simulink model "Shanthan_Heeirthan_EE469S3D_R45 (1)"  (R2023a)
settings: Solver=FixedStepDiscrete  StartTime=0.0  StopTime=120  FixedStep=dt0  RelTol=1e-3  EnableMultiTasking=on
PostLoadFcn:
  | %Set the size for the model
  | set_param(gcs,'Location',[10 10 1270 970])
  | %Set the zoom factor for the model
  | set_param(gcs,'ZoomFactor','100')
InitFcn:
  | tic
  | % Students Add call to their M-file HERE
  | Shanthan_Heeirthan_EE460_Final
  | INIT_S3D_01
StartFcn:
  | tend0=toc;
  | tic;
StopFcn:
  | tend=toc;
  | disp(['Simulation time = ' num2str(tout(end)) ' sec'])
  | disp(['Real time = ' num2str(tend) ' sec'])
  | title('DONE')
  | SCORE=round((max(0,120-tout(end)-tend0))*4+10*(40-FuelBurned)+sum(100*double(PDONE)-100*double(PDONE<.5)));
  | PlotS3D(PlotInput);
  | text(15,22,['S: ' num2str(SCORE)]);
values from neighbouring files (symbols this model uses):
  A = [0 1 0 0 0 0 ... (first row only)    [Shanthan_Heeirthan_EE460_Final (1).m]
  B = [0 0 0 ... (first row only)    [Shanthan_Heeirthan_EE460_Final (1).m]
  bm = [1 1 -1 -1 0 0 0 0; 0 0 0 0 -1 1 1 -1; -1 1 -1 1 3 -3 3 -3]    [Shanthan_Heeirthan_EE460_Final (1).m]
  C = [1 0 0 0 0 0 ... (first row only)    [Shanthan_Heeirthan_EE460_Final (1).m]
  D = [0 0 0 ... (first row only)    [Shanthan_Heeirthan_EE460_Final (1).m]
  Denchptheta = TFchptheta.Den{1}    [Shanthan_Heeirthan_EE460_Final (1).m]
  Denchpxy = TFchpxy.Den{1}    [Shanthan_Heeirthan_EE460_Final (1).m]
  Denclptheta = TFclptheta.Den{1}    [Shanthan_Heeirthan_EE460_Final (1).m]
  Denclpxy = TFclpxy.Den{1}    [Shanthan_Heeirthan_EE460_Final (1).m]
  Denlp = TFlp.Den{1}    [Shanthan_Heeirthan_EE460_Final (1).m]
  Kd = 2.1+0    (= 2.1)    [Shanthan_Heeirthan_EE460_Final (1).m]
  Ki = 0.0001    [Shanthan_Heeirthan_EE460_Final (1).m]
  Kp = 1.1+0.2    (= 1.3)    [Shanthan_Heeirthan_EE460_Final (1).m]
  L = place(A',C',ep)'    [Shanthan_Heeirthan_EE460_Final (1).m]
  Numchptheta = TFchptheta.Num{1}    [Shanthan_Heeirthan_EE460_Final (1).m]
  Numchpxy = TFchpxy.Num{1}    [Shanthan_Heeirthan_EE460_Final (1).m]
  Numclptheta = TFclptheta.Num{1}    [Shanthan_Heeirthan_EE460_Final (1).m]
  Numclpxy = TFclpxy.Num{1}    [Shanthan_Heeirthan_EE460_Final (1).m]
  Numlp = TFlp.Num{1}    [Shanthan_Heeirthan_EE460_Final (1).m]
  Pnewdata = [LVL.P1 LVL.P2 LVL.P3 LVL.P4]    [Shanthan_Heeirthan_EE460_Final (1).m]
  Sconfig = 1    [Shanthan_Heeirthan_EE460_Final (1).m]
  TFP1 = 2    [Shanthan_Heeirthan_EE460_Final (1).m]
  TFP1z = 1    [Shanthan_Heeirthan_EE460_Final (1).m]
  TFP2 = 2    [Shanthan_Heeirthan_EE460_Final (1).m]
  TFP2z = 1    [Shanthan_Heeirthan_EE460_Final (1).m]
  TFP3 = 2    [Shanthan_Heeirthan_EE460_Final (1).m]
  TFP3z = 1    [Shanthan_Heeirthan_EE460_Final (1).m]
  TFP4 = 2    [Shanthan_Heeirthan_EE460_Final (1).m]
  TFP4z = 1    [Shanthan_Heeirthan_EE460_Final (1).m]
  wcf = 2    [Shanthan_Heeirthan_EE460_Final (1).m]
  wcft = 10    [Shanthan_Heeirthan_EE460_Final (1).m]
undefined symbols (not defined in the file or in its folder): d2r, DiscIntNeverNeededParam, dt, dt0, fr, HM_S, HM_U, J, Jbase, JC0, L13, L24, LVL, M, M1, M2, M3, M4, mdti, Pdata, PTvec, r2d, SLIM, SQ, SSF, TOLdata, ULIM
libraries: simulink x85, aerolibanimutils x1, matrix_library x1
(part 2 of 7)

== system Shanthan_Heeirthan_EE469S3D_R45 (1)/S3D_Plant/Sensors/CASE1 ==
  X : Inport
  Action Port : ActionPort  ActionPortLabel=case [ 1 ]:
  Constant2 : Constant  Value=SSF  SampleTime=dt0
  Gain : Gain
  Mux{,1..3} (4 alike) : Mux  Inputs=3
  Product : Product
  THTaccel : Subsystem
  THTpos1 : Subsystem
  THTvel : Subsystem
  Xaccel : Subsystem
  Xpos1 : Subsystem
  Xvel : Subsystem
  Yaccel : Subsystem
  Ypos1 : Subsystem
  Yvel : Subsystem
  Out1 : Outport
  wires:
  Constant2/1 -> Product/2
  Product/1 -> Gain/1
  Mux3/1 -> Product/1
  Gain/1 -> Out1/1
  THTaccel/1(thtddt1) -> Mux2/3
  THTvel/1(thtdt1) -> Mux2/2
  THTpos1/1(tht1) -> Mux2/1
  Mux2/1 -> Mux3/3
  Yaccel/1(yddt1) -> Mux1/3
  Yvel/1(ydt1) -> Mux1/2
  Ypos1/1(y1) -> Mux1/1
  Mux1/1 -> Mux3/2
  Mux/1 -> Mux3/1
  Xaccel/1(xddt1) -> Mux/3
  Xpos1/1(x1) -> Mux/1
  Xvel/1(xdt1) -> Mux/2
  X/1 -> Xpos1/1(X), Xvel/1(X), Xaccel/1(X), Ypos1/1(X), Yvel/1(X), Yaccel/1(X), THTpos1/1(X), THTvel/1(X), THTaccel/1(X)

== system Shanthan_Heeirthan_EE469S3D_R45 (1)/S3D_Plant/Sensors/CASE2 ==
  X : Inport
  Action Port : ActionPort  ActionPortLabel=case [ 2 ]:
  Constant2 : Constant  Value=SSF([1 1 2 4 4 5 7 7 8])  SampleTime=dt0
  Gain : Gain
  Mux{,1..3} (4 alike) : Mux  Inputs=3
  Product : Product
  THTpos1 : Subsystem
  THTpos2 : Subsystem
  THTvel : Subsystem
  Xpos1 : Subsystem
  Xpos2 : Subsystem
  Xvel : Subsystem
  Ypos1 : Subsystem
  Ypos2 : Subsystem
  Yvel : Subsystem
  Out1 : Outport
  wires:
  Constant2/1 -> Product/2
  Product/1 -> Gain/1
  Mux3/1 -> Product/1
  Gain/1 -> Out1/1
  X/1 -> THTvel/1(X), THTpos2/1(X), THTpos1/1(X), Yvel/1(X), Ypos2/1(X), Ypos1/1(X), Xvel/1(X), Xpos2/1(X), Xpos1/1(X)
  Xpos2/1(x1) -> Mux/2
  Xpos1/1(x1) -> Mux/1
  Xvel/1(xdt1) -> Mux/3
  Mux/1 -> Mux3/1
  Mux1/1 -> Mux3/2
  Ypos1/1(y1) -> Mux1/1
  Ypos2/1(y1) -> Mux1/2
  Yvel/1(ydt1) -> Mux1/3
  Mux2/1 -> Mux3/3
  THTpos1/1(tht1) -> Mux2/1
  THTpos2/1(tht1) -> Mux2/2
  THTvel/1(thtdt1) -> Mux2/3

== system Shanthan_Heeirthan_EE469S3D_R45 (1)/S3D_Plant/Sensors/CASE3 ==
  X : Inport
  Action Port : ActionPort  ActionPortLabel=default:
  Constant2 : Constant  Value=SSF([1 1 1 4 4 4 7 7 7])  SampleTime=dt0
  Gain : Gain
  Mux{,1..3} (4 alike) : Mux  Inputs=3
  Product : Product
  THTpos1 : Subsystem
  THTpos2 : Subsystem
  THTpos3 : Subsystem
  Xpos1 : Subsystem
  Xpos2 : Subsystem
  Xpos3 : Subsystem
  Ypos1 : Subsystem
  Ypos2 : Subsystem
  Ypos3 : Subsystem
  Out1 : Outport
  wires:
  Constant2/1 -> Product/2
  Product/1 -> Gain/1
  Mux3/1 -> Product/1
  Gain/1 -> Out1/1
  THTpos3/1(tht1) -> Mux2/3
  THTpos2/1(tht1) -> Mux2/2
  THTpos1/1(tht1) -> Mux2/1
  Mux2/1 -> Mux3/3
  Ypos3/1(y1) -> Mux1/3
  Ypos2/1(y1) -> Mux1/2
  Ypos1/1(y1) -> Mux1/1
  Mux1/1 -> Mux3/2
  Mux/1 -> Mux3/1
  Xpos3/1(xddt1) -> Mux/3
  Xpos1/1(x1) -> Mux/1
  Xpos2/1(xdt1) -> Mux/2
  X/1 -> Xpos1/1(X), Ypos1/1(X), THTpos1/1(X), THTpos2/1(X), THTpos3/1(X), Ypos3/1(X), Ypos2/1(X), Xpos3/1(X), Xpos2/1(X)

== system Shanthan_Heeirthan_EE469S3D_R45 (1)/S3D_Plant/Sensors/ConvertINT16 ==
  SDouble : Inport
  Bus Creator : BusCreator  Inputs=9
  Data Type Conversion{,1..8} (9 alike) : DataTypeConversion  OutDataTypeStr=int16  SampleTime=dt0  SaturateOnIntegerOverflow=off  RndMeth=Floor
  Demux : Demux  Outputs=9
  INT16 : Outport
  wires:
  Data Type Conversion8/1 -> Bus Creator/9  "Sensor9"
  Data Type Conversion7/1 -> Bus Creator/8  "Sensor8"
  Data Type Conversion6/1 -> Bus Creator/7  "Sensor7"
  Data Type Conversion5/1 -> Bus Creator/6  "Sensor6"
  Data Type Conversion4/1 -> Bus Creator/5  "Sensor5"
  Data Type Conversion3/1 -> Bus Creator/4  "Sensor4"
  Data Type Conversion2/1 -> Bus Creator/3  "Sensor3"
  Demux/5 -> Data Type Conversion4/1
  Demux/3 -> Data Type Conversion2/1
  Demux/6 -> Data Type Conversion5/1
  Demux/4 -> Data Type Conversion3/1
  Demux/9 -> Data Type Conversion8/1
  Demux/7 -> Data Type Conversion6/1
  Demux/8 -> Data Type Conversion7/1
  SDouble/1 -> Demux/1
  Data Type Conversion1/1 -> Bus Creator/2  "Sensor2"
  Bus Creator/1 -> INT16/1  "INT16"
  Demux/1 -> Data Type Conversion/1
  Demux/2 -> Data Type Conversion1/1
  Data Type Conversion/1 -> Bus Creator/1  "Sensor1"

== system Shanthan_Heeirthan_EE469S3D_R45 (1)/S3D_Plant/Sensors/HealthMonitoring ==
  SensorValues : Inport
  Bus Creator1 : BusCreator  Inputs=18
  Bus Selector1 : BusSelector  OutputSignals=Sensor1,Sensor2,Sensor3,Sensor4,Sensor5,Sensor6,Sensor7,Sensor8,Sensor9
  Bus Selector2 : BusSelector  OutputSignals=Sensor1,Sensor2,Sensor3,Sensor4,Sensor5,Sensor6,Sensor7,Sensor8,Sensor9
  Subsystem : Subsystem
  Subsystem1 : Subsystem
  Subsystem2 : Subsystem
  Subsystem3 : Subsystem
  Subsystem4 : Subsystem
  Subsystem5 : Subsystem
  Subsystem6 : Subsystem
  Subsystem7 : Subsystem
  Subsystem8 : Subsystem
  Sensors : Outport
  wires:
  Bus Creator1/1 -> Sensors/1  "Sensors"
  Bus Selector2/4 -> Bus Creator1/4  "<Sensor4>"
  Bus Selector2/8 -> Bus Creator1/8  "<Sensor8>"
  Bus Selector2/6 -> Bus Creator1/6  "<Sensor6>"
  Bus Selector2/5 -> Bus Creator1/5  "<Sensor5>"
  Bus Selector2/3 -> Bus Creator1/3  "<Sensor3>"
  Bus Selector2/9 -> Bus Creator1/9  "<Sensor9>"
  Bus Selector2/2 -> Bus Creator1/2  "<Sensor2>"
  Bus Selector2/1 -> Bus Creator1/1  "<Sensor1>"
  Bus Selector2/7 -> Bus Creator1/7  "<Sensor7>"
  SensorValues/1 -> Bus Selector1/1, Bus Selector2/1
  Subsystem/1(Out1) -> Bus Creator1/10  "S1fail"
  Bus Selector1/8 -> Subsystem7/1(In1)  "<Sensor8>"
  Bus Selector1/3 -> Subsystem2/1(In1)  "<Sensor3>"
  Bus Selector1/7 -> Subsystem6/1(In1)  "<Sensor7>"
  Bus Selector1/2 -> Subsystem1/1(In1)  "<Sensor2>"
  Subsystem2/1(Out1) -> Bus Creator1/12  "S3fail"
  Subsystem1/1(Out1) -> Bus Creator1/11  "S2fail"
  Bus Selector1/6 -> Subsystem5/1(In1)  "<Sensor6>"
  Subsystem3/1(Out1) -> Bus Creator1/13  "S4fail"
  Bus Selector1/4 -> Subsystem3/1(In1)  "<Sensor4>"
  Bus Selector1/5 -> Subsystem4/1(In1)  "<Sensor5>"
  Bus Selector1/9 -> Subsystem8/1(In1)  "<Sensor9>"
  Subsystem5/1(Out1) -> Bus Creator1/15  "S6fail"
  Subsystem4/1(Out1) -> Bus Creator1/14  "S5fail"
  Subsystem6/1(Out1) -> Bus Creator1/16  "S7fail"
  Subsystem8/1(Out1) -> Bus Creator1/18  "S9fail"
  Subsystem7/1(Out1) -> Bus Creator1/17  "S8fail"
  Bus Selector1/1 -> Subsystem/1(In1)  "<Sensor1>"

== system Shanthan_Heeirthan_EE469S3D_R45 (1)/S3D_Plant/ThrusterValues/FailModes ==
  Ucmd : Inport
  MP : Inport  Port=2
  Bus Creator : BusCreator  Inputs=10
  Ufail1 : Subsystem  mask{Udx=1, Tank=1}
      mask prompts: Udx "Input Index of U (1-8)"; Tank "Input Fuel Tank (1-4)"
  Ufail10 : Subsystem  mask{Udx=10, Tank=1}
      mask prompts: Udx "Input Index of U (1-8)"; Tank "Input Fuel Tank (1-4)"
  Ufail2 : Subsystem  mask{Udx=2, Tank=2}
      mask prompts: Udx "Input Index of U (1-8)"; Tank "Input Fuel Tank (1-4)"
  Ufail3 : Subsystem  mask{Udx=3, Tank=3}
      mask prompts: Udx "Input Index of U (1-8)"; Tank "Input Fuel Tank (1-4)"
  Ufail4 : Subsystem  mask{Udx=4, Tank=4}
      mask prompts: Udx "Input Index of U (1-8)"; Tank "Input Fuel Tank (1-4)"
  Ufail5 : Subsystem  mask{Udx=5, Tank=1}
      mask prompts: Udx "Input Index of U (1-8)"; Tank "Input Fuel Tank (1-4)"
  Ufail6 : Subsystem  mask{Udx=6, Tank=2}
      mask prompts: Udx "Input Index of U (1-8)"; Tank "Input Fuel Tank (1-4)"
  Ufail7 : Subsystem  mask{Udx=7, Tank=3}
      mask prompts: Udx "Input Index of U (1-8)"; Tank "Input Fuel Tank (1-4)"
  Ufail8 : Subsystem  mask{Udx=8, Tank=4}
      mask prompts: Udx "Input Index of U (1-8)"; Tank "Input Fuel Tank (1-4)"
  Ufail9 : Subsystem  mask{Udx=9, Tank=1}
      mask prompts: Udx "Input Index of U (1-8)"; Tank "Input Fuel Tank (1-4)"
  U : Outport
  wires:
  Bus Creator/1 -> U/1  "U"
  Ufail7/1(Uout) -> Bus Creator/7  "U7"
  Ufail6/1(Uout) -> Bus Creator/6  "U6"
  Ufail8/1(Uout) -> Bus Creator/8  "U8"
  Ufail9/1(Uout) -> Bus Creator/9  "U9"
  Ufail10/1(Uout) -> Bus Creator/10  "U10"
  Ufail5/1(Uout) -> Bus Creator/5  "U5"
  Ufail4/1(Uout) -> Bus Creator/4  "U4"
  Ufail3/1(Uout) -> Bus Creator/3  "U3"
  Ufail2/1(Uout) -> Bus Creator/2  "U2"
  Ufail1/1(Uout) -> Bus Creator/1  "U1"
  MP/1 -> Ufail1/2(MP), Ufail3/2(MP), Ufail4/2(MP), Ufail8/2(MP), Ufail7/2(MP), Ufail6/2(MP), Ufail5/2(MP), Ufail2/2(MP)
  Ucmd/1 -> Ufail1/1(Uin), Ufail4/1(Uin), Ufail9/1(Uin), Ufail10/1(Uin), Ufail8/1(Uin), Ufail7/1(Uin), Ufail6/1(Uin), Ufail5/1(Uin), Ufail3/1(Uin), Ufail2/1(Uin)

== system Shanthan_Heeirthan_EE469S3D_R45 (1)/S3D_Plant/ThrusterValues/HealthMonitoring ==
  Uvalues : Inport
  UCMD : Inport  Port=2
  Bus Creator2 : BusCreator  Inputs=20
  Bus Selector10 : BusSelector  OutputSignals=U1,U2,U3,U4,U5,U6,U7,U8,U9,U10
  Bus Selector11 : BusSelector  OutputSignals=U1fail,U2fail,U3fail,U4fail,U5fail,U6fail,U7fail,U8fail,U9fail,U10fail
  DetectFailures : Subsystem
  U : Outport
  wires:
  Bus Selector10/1 -> Bus Creator2/1  "<U1>"
  Bus Selector10/2 -> Bus Creator2/2  "<U2>"
  Bus Selector10/9 -> Bus Creator2/9  "<U9>"
  Bus Selector10/5 -> Bus Creator2/5  "<U5>"
  Bus Selector10/3 -> Bus Creator2/3  "<U3>"
  Bus Selector10/6 -> Bus Creator2/6  "<U6>"
  Bus Selector10/7 -> Bus Creator2/7  "<U7>"
  Bus Selector10/8 -> Bus Creator2/8  "<U8>"
  Bus Selector10/4 -> Bus Creator2/4  "<U4>"
  Bus Selector10/10 -> Bus Creator2/10  "<U10>"
  Bus Creator2/1 -> U/1  "U"
  Bus Selector11/1 -> Bus Creator2/11  "<U1fail>"
  Bus Selector11/2 -> Bus Creator2/12  "<U2fail>"
  Bus Selector11/3 -> Bus Creator2/13  "<U3fail>"
  Bus Selector11/4 -> Bus Creator2/14  "<U4fail>"
  Bus Selector11/5 -> Bus Creator2/15  "<U5fail>"
  Bus Selector11/6 -> Bus Creator2/16  "<U6fail>"
  Bus Selector11/7 -> Bus Creator2/17  "<U7fail>"
  Bus Selector11/8 -> Bus Creator2/18  "<U8fail>"
  Bus Selector11/9 -> Bus Creator2/19  "<U9fail>"
  Bus Selector11/10 -> Bus Creator2/20  "<U10fail>"
  UCMD/1 -> DetectFailures/2(UCMD)
  Uvalues/1 -> DetectFailures/1(Uvalues), Bus Selector10/1
  DetectFailures/1(Out2) -> Bus Selector11/1

== system Shanthan_Heeirthan_EE469S3D_R45 (1)/control_law/CMD/CMDprocess ==
  Y_IN : Inport
  Bus Selector : BusSelector  OutputSignals=Y_IN_sens.X1_m,Y_IN_sens.Y_m  OutputAsBus=on
  CommandTypes : Subsystem
  Constant : Constant
  Constant3 : Constant  Value=Pnewdata
  Selector1 : Selector  NumberOfDimensions=2  InputPortWidth=3  IndexOptions=Select all,Index vector (port)  Indices=[1 3],1  OutputSizes=1,1
  CMD : Outport
  wires:
  Constant3/1 -> Selector1/1  "Pdata"
  Y_IN/1 -> Bus Selector/1
  Selector1/1 -> CommandTypes/1(Pdata)  "CMDS"
  CommandTypes/1(CMDS) -> CMD/1
  Constant/1 -> Selector1/2, CommandTypes/2(Point)  "Point"
  Bus Selector/1 -> CommandTypes/3(Sensed)  "Sensed"

== system Shanthan_Heeirthan_EE469S3D_R45 (1)/control_law/InputDataConditioning/SensorConditioning ==
  Y_BUS : Inport
  Bus Creator : BusCreator  Inputs=9
  Bus Selector : BusSelector  OutputSignals=S1fail,S2fail,S3fail,Sensor1,Sensor2,Sensor3  OutputAsBus=on
  Bus Selector1 : BusSelector  OutputSignals=S4fail,S5fail,S6fail,Sensor4,Sensor5,Sensor6  OutputAsBus=on
  Bus Selector2 : BusSelector  OutputSignals=Sensor7,Sensor8,Sensor9,S7fail,S8fail,S9fail  OutputAsBus=on
  JustX : Subsystem
  JustY : Subsystem
  JustZ : Subsystem
  Y_sens : Outport
  wires:
  Y_BUS/1 -> Bus Selector2/1, Bus Selector/1, Bus Selector1/1
  Bus Selector/1 -> JustX/1(Xsens)  "Sensors"
  Bus Selector1/1 -> JustY/1(Ysens)  "Sensors"
  Bus Selector2/1 -> JustZ/1(Zsens)  "Sensors"
  JustX/1(xpos) -> Bus Creator/1  "X1_m"
  Bus Creator/1 -> Y_sens/1  "Y_IN_sens"
  JustX/2(xvel) -> Bus Creator/2  "X_mps"
  JustX/3(xacc) -> Bus Creator/3  "X_mps2"
  JustY/1(ypos) -> Bus Creator/4  "Y_m"
  JustY/2(yvel) -> Bus Creator/5  "Y_mps"
  JustY/3(yacc) -> Bus Creator/6  "Y_mps2"
  JustZ/1(thetapos) -> Bus Creator/7  "theta_deg"
  JustZ/2(thetavel) -> Bus Creator/8  "theta_degps"
  JustZ/3(thetaacc) -> Bus Creator/9  "theta_degps2"

== system Shanthan_Heeirthan_EE469S3D_R45 (1)/control_law/InputDataConditioning/xhatsel ==
  xhat : Inport
  Bus Creator1 : BusCreator  Inputs=6
  Demux : Demux  Outputs=6
  Gain : Gain  Gain=180/pi
  Gain1 : Gain  Gain=180/pi
  x_hat : Outport
  wires:
  xhat/1 -> Demux/1
  Demux/4 -> Bus Creator1/4  "y_vel_est_mps"
  Bus Creator1/1 -> x_hat/1  "x_hat"
  Demux/2 -> Bus Creator1/2  "x_vel_est_mps"
  Demux/3 -> Bus Creator1/3  "y_pos_est_m"
  Demux/1 -> Bus Creator1/1  "x_pos_est_m"
  Demux/6 -> Gain1/1  "theta_vel_est_radps"
  Gain1/1 -> Bus Creator1/6  "theta_vel_est_degps"
  Demux/5 -> Gain/1  "theta_pos_est_rad"
  Gain/1 -> Bus Creator1/5  "theta_pos_est_deg"

== system Shanthan_Heeirthan_EE469S3D_R45 (1)/control_law/Regulator/CompX ==
  Y_IN : Inport
  Bus Creator : BusCreator  Inputs=2
  Bus Selector : BusSelector  OutputSignals=Y_IN_sens.X1_m,Y_IN_sens.X_mps,Y_IN_sens.X_mps2
  Discrete Transfer Fcn : DiscreteTransferFcn  Numerator=Numclpxy  Denominator=Denclpxy  SampleTime=dt
  Discrete Transfer Fcn1 : DiscreteTransferFcn  Numerator=Numchpxy  Denominator=Denchpxy  SampleTime=dt
  Discrete Transfer Fcn2 : DiscreteTransferFcn  Numerator=Numchpxy  Denominator=Denchpxy  SampleTime=dt
  Gain : Gain  Gain=wcf
  Sum : Sum  Inputs=|++
  Sum1 : Sum  Inputs=|++
  X_filt : Outport
  wires:
  Y_IN/1 -> Bus Selector/1
  Bus Selector/1 -> Discrete Transfer Fcn/1  "<X1_m>"
  Bus Selector/2 -> Discrete Transfer Fcn1/1  "<X_mps>"
  Bus Selector/3 -> Discrete Transfer Fcn2/1  "<X_mps2>"
  Sum1/1 -> Bus Creator/2  "X_mps"
  Gain/1 -> Sum1/1
  Discrete Transfer Fcn/1 -> Sum/1
  Discrete Transfer Fcn1/1 -> Sum/2, Gain/1
  Discrete Transfer Fcn2/1 -> Sum1/2
  Sum/1 -> Bus Creator/1  "X1_m"
  Bus Creator/1 -> X_filt/1

== system Shanthan_Heeirthan_EE469S3D_R45 (1)/control_law/Regulator/CompY ==
  Y_IN : Inport
  Bus Creator : BusCreator  Inputs=2
  Bus Selector : BusSelector  OutputSignals=Y_IN_sens.Y_m,Y_IN_sens.Y_mps,Y_IN_sens.Y_mps2
  Discrete Transfer Fcn : DiscreteTransferFcn  Numerator=Numclpxy  Denominator=Denclpxy  SampleTime=dt
  Discrete Transfer Fcn1 : DiscreteTransferFcn  Numerator=Numchpxy  Denominator=Denchpxy  SampleTime=dt
  Discrete Transfer Fcn2 : DiscreteTransferFcn  Numerator=Numchpxy  Denominator=Denchpxy  SampleTime=dt
  Gain : Gain  Gain=wcf
  Sum : Sum  Inputs=|++
  Sum1 : Sum  Inputs=|++
  Y_filt : Outport
  wires:
  Bus Creator/1 -> Y_filt/1
  Sum/1 -> Bus Creator/1  "Y_m"
  Discrete Transfer Fcn2/1 -> Sum1/2
  Discrete Transfer Fcn1/1 -> Gain/1, Sum/2
  Discrete Transfer Fcn/1 -> Sum/1
  Gain/1 -> Sum1/1
  Sum1/1 -> Bus Creator/2  "Y_mps"
  Bus Selector/3 -> Discrete Transfer Fcn2/1  "<Y_mps2>"
  Bus Selector/2 -> Discrete Transfer Fcn1/1  "<Y_mps>"
  Bus Selector/1 -> Discrete Transfer Fcn/1  "<Y_m>"
  Y_IN/1 -> Bus Selector/1

== system Shanthan_Heeirthan_EE469S3D_R45 (1)/control_law/Regulator/Comptheta ==
  Y_IN : Inport
  Bus Creator : BusCreator  Inputs=2
  Bus Selector : BusSelector  OutputSignals=Y_IN_sens.theta_deg,Y_IN_sens.theta_degps,Y_IN_sens.theta_degps2
  Discrete Transfer Fcn : DiscreteTransferFcn  Numerator=Numclptheta  Denominator=Denclptheta  SampleTime=dt
  Discrete Transfer Fcn1 : DiscreteTransferFcn  Numerator=Numchptheta  Denominator=Denchptheta  SampleTime=dt
  Discrete Transfer Fcn2 : DiscreteTransferFcn  Numerator=Numchptheta  Denominator=Denchptheta  SampleTime=dt
  Gain : Gain  Gain=wcft
  Sum : Sum  Inputs=|++
  Sum1 : Sum  Inputs=|++
  theta_filt : Outport
  wires:
  Bus Creator/1 -> theta_filt/1
  Sum/1 -> Bus Creator/1  "theta_deg"
  Discrete Transfer Fcn2/1 -> Sum1/2
  Discrete Transfer Fcn1/1 -> Gain/1, Sum/2
  Discrete Transfer Fcn/1 -> Sum/1
  Gain/1 -> Sum1/1
  Sum1/1 -> Bus Creator/2  "theta_degps"
  Bus Selector/3 -> Discrete Transfer Fcn2/1  "<theta_degps2>"
  Bus Selector/2 -> Discrete Transfer Fcn1/1  "<theta_degps>"
  Bus Selector/1 -> Discrete Transfer Fcn/1  "<theta_deg>"
  Y_IN/1 -> Bus Selector/1

== system Shanthan_Heeirthan_EE469S3D_R45 (1)/control_law/Regulator/MassVariable ==
  Ulim : Inport
  Bus Creator : BusCreator  Inputs=10
  Bus to Vector : BusToVector
  Constant : Constant  Value=M
  Demux : Demux  Outputs=10
  Discrete-Time Integrator : DiscreteIntegrator  SampleTime=-1  ICPrevOutput=DiscIntNeverNeededParam  ICPrevScaledInput=DiscIntNeverNeededParam
  Gain : Gain  Gain=mdti
  Sum : Sum  Inputs=+
  Sum1 : Sum  Inputs=|+-
  Mass : Outport
  wires:
  Ulim/1 -> Demux/1
  Demux/1 -> Bus Creator/1  "U1cmd"
  Demux/2 -> Bus Creator/2  "U2cmd"
  Demux/3 -> Bus Creator/3  "U3cmd"
  Demux/4 -> Bus Creator/4  "U4cmd"
  Demux/5 -> Bus Creator/5  "U5cmd"
  Demux/6 -> Bus Creator/6  "U6cmd"
  Demux/7 -> Bus Creator/7  "U7cmd"
  Demux/8 -> Bus Creator/8  "U8cmd"
  Demux/9 -> Bus Creator/9  "U9cmd"
  Demux/10 -> Bus Creator/10  "U10cmd"
  Bus Creator/1 -> Bus to Vector/1
  Bus to Vector/1 -> Gain/1
  Gain/1 -> Discrete-Time Integrator/1  "mdot"
  Discrete-Time Integrator/1 -> Sum/1  "mchanged"
  Sum/1 -> Sum1/2
  Constant/1 -> Sum1/1  "realm"
  Sum1/1 -> Mass/1  "Mass"

== system Shanthan_Heeirthan_EE469S3D_R45 (1)/control_law/thrustercmd/CAcreator ==
  DCM : Inport
  U_lim : Inport  Port=2
  Bus Creator : BusCreator  Inputs=10
  Bus Creator1 : BusCreator  Inputs=8
  Bus Selector : BusSelector  OutputSignals=U1cmd,U2cmd,U3cmd,U4cmd,U5cmd,U6cmd,U7cmd,U8cmd
  Constant : Constant  Value=bm
  Demux1 : Demux  Outputs=10
  Matrix Multiply : Product  Multiplication=Matrix(*)
  Matrix Multiply1 : Product  Multiplication=Matrix(*)
  Transpose : Math  Operator=transpose
  CAout : Outport
  wires:
  Demux1/4 -> Bus Creator/4  "U4cmd"
  Bus Selector/5 -> Bus Creator1/5  "<U5cmd>"
  Demux1/7 -> Bus Creator/7  "U7cmd"
  Bus Selector/2 -> Bus Creator1/2  "<U2cmd>"
  Bus Selector/3 -> Bus Creator1/3  "<U3cmd>"
  Demux1/9 -> Bus Creator/9  "U9cmd"
  Demux1/5 -> Bus Creator/5  "U5cmd"
  Demux1/2 -> Bus Creator/2  "U2cmd"
  Demux1/1 -> Bus Creator/1  "U1cmd"
  Demux1/8 -> Bus Creator/8  "U8cmd"
  Bus Selector/4 -> Bus Creator1/4  "<U4cmd>"
  Demux1/10 -> Bus Creator/10  "U10cmd"
  Demux1/3 -> Bus Creator/3  "U3cmd"
  Bus Creator/1 -> Bus Selector/1  "Ulim"
  Bus Selector/7 -> Bus Creator1/7  "<U7cmd>"
  Bus Selector/1 -> Bus Creator1/1  "<U1cmd>"
  Demux1/6 -> Bus Creator/6  "U6cmd"
  Bus Selector/6 -> Bus Creator1/6  "<U6cmd>"
  Bus Selector/8 -> Bus Creator1/8  "<U8cmd>"
  U_lim/1 -> Demux1/1
  Constant/1 -> Matrix Multiply/1  "bm"
  Bus Creator1/1 -> Matrix Multiply/2  "Ulim"
  Matrix Multiply1/1 -> CAout/1  "CAout"
  Matrix Multiply/1 -> Matrix Multiply1/2  "CAout"
  DCM/1 -> Transpose/1
  Transpose/1 -> Matrix Multiply1/1

== system Shanthan_Heeirthan_EE469S3D_R45 (1)/control_law/thrustercmd/DCM ==
  Y_IN : Inport
  Bus Selector : BusSelector  OutputSignals=Y_IN_sens.theta_deg
  Constant : Constant  Value=[0 0 0;0 0 0;0 0 1]
  Cos : Trigonometry  Operator=cos
  Gain : Gain  Gain=pi/180
  Gain1 : Gain  Gain=[1 0 0; 0 1 0; 0 0 0]
  Gain2 : Gain  Gain=[0 -1 0;1 0 0;0 0 0]
  Sin : Trigonometry
  Sum : Sum  Inputs=|++
  Sum1 : Sum  Inputs=|++
  Transpose : Math  Operator=transpose
  IUR : Outport
  wires:
  Y_IN/1 -> Bus Selector/1
  Bus Selector/1 -> Gain/1  "<theta_deg>"
  Gain/1 -> Cos/1, Sin/1
  Cos/1 -> Gain1/1
  Sin/1 -> Gain2/1
  Gain1/1 -> Sum/1
  Gain2/1 -> Sum/2
  Sum/1 -> Sum1/1
  Constant/1 -> Sum1/2
  Sum1/1 -> Transpose/1
  Transpose/1 -> IUR/1

== system Shanthan_Heeirthan_EE469S3D_R45 (1)/control_law/thrustercmd/GenInverse ==
  Ufail : Inport
  Constant : Constant  Value=bm
  Constant2 : Constant  Value=bm
  Divide : Product  Inputs=/  Multiplication=Matrix(*)
  Divide1 : Product  Inputs=/  Multiplication=Matrix(*)
  Divide2 : Product  Inputs=/  Multiplication=Matrix(*)
  Gain : Gain  Gain=2
  Matrix Multiply{,1..3} (4 alike) : Product  Multiplication=Matrix(*)
  Transpose{,1..3} (4 alike) : Math  Operator=transpose
  WeightedMatrix : Subsystem
  ginv : Outport
  wires:
  WeightedMatrix/1(Weight) -> Transpose2/1, Transpose/1
  Transpose/1 -> Divide/1
  Constant/1 -> Matrix Multiply1/1, Transpose1/1
  Divide/1 -> Matrix Multiply/1
  Transpose1/1 -> Matrix Multiply/2
  Transpose2/1 -> Divide1/1
  Divide1/1 -> Matrix Multiply1/2
  Matrix Multiply1/1 -> Matrix Multiply2/1
  Matrix Multiply2/1 -> Divide2/1
  Matrix Multiply/1 -> Matrix Multiply3/1
  Divide2/1 -> Matrix Multiply3/2
  Constant2/1 -> Transpose3/1
  Transpose3/1 -> Matrix Multiply2/2
  Matrix Multiply3/1 -> Gain/1  "pinv"
  Gain/1 -> ginv/1  "ginv"
  Ufail/1 -> WeightedMatrix/1(Ufail)

== system Shanthan_Heeirthan_EE469S3D_R45 (1)/S3D_Plant/Comm/P1/DirectionCompensation2 ==
  In1 : Inport
  Compare To Constant : simulink/Logic and Bit Operations/Compare To Constant  relop=<=  const=pi  OutDataTypeStr=boolean
  Compare To Constant1 : simulink/Logic and Bit Operations/Compare To Constant  relop=>=  const=-pi  OutDataTypeStr=boolean
  Constant1 : Constant  Value=2*pi  SampleTime=dt0
  Constant2 : Constant  Value=2*pi  SampleTime=dt0
  Constant3 : Constant  Value=2*pi  SampleTime=dt0
  Mod : Math  Operator=mod
  Sum : Sum  Inputs=|+-
  Sum1 : Sum  Inputs=|++
  Switch : Switch  Criteria=u2 > Threshold  SaturateOnIntegerOverflow=off  InputSameDT=off
  Switch1 : Switch  SaturateOnIntegerOverflow=off  InputSameDT=off
  Switch2 : Switch  Criteria=u2 > Threshold  SaturateOnIntegerOverflow=off  InputSameDT=off
  Out1 : Outport
  wires:
  Sum1/1 -> Switch2/3
  Switch2/1 -> Switch1/3
  Compare To Constant1/1 -> Switch2/2
  Switch/1 -> Switch1/1
  Sum/1 -> Switch/3
  Compare To Constant/1 -> Switch/2
  Mod/1 -> Compare To Constant/1, Sum/1, Switch1/2, Switch2/1, Compare To Constant1/1, Sum1/1, Switch/1
  Switch1/1 -> Out1/1  "Mod_rad"
  Constant2/1 -> Sum1/2
  Constant1/1 -> Sum/2
  In1/1 -> Mod/1
  Constant3/1 -> Mod/2

== system Shanthan_Heeirthan_EE469S3D_R45 (1)/S3D_Plant/Comm/P2/DirectionCompensation2 ==
  In1 : Inport
  Compare To Constant : simulink/Logic and Bit Operations/Compare To Constant  relop=<=  const=pi  OutDataTypeStr=boolean
  Compare To Constant1 : simulink/Logic and Bit Operations/Compare To Constant  relop=>=  const=-pi  OutDataTypeStr=boolean
  Constant1 : Constant  Value=2*pi  SampleTime=dt0
  Constant2 : Constant  Value=2*pi  SampleTime=dt0
  Constant3 : Constant  Value=2*pi  SampleTime=dt0
  Mod : Math  Operator=mod
  Sum : Sum  Inputs=|+-
  Sum1 : Sum  Inputs=|++
  Switch : Switch  Criteria=u2 > Threshold  SaturateOnIntegerOverflow=off  InputSameDT=off
  Switch1 : Switch  SaturateOnIntegerOverflow=off  InputSameDT=off
  Switch2 : Switch  Criteria=u2 > Threshold  SaturateOnIntegerOverflow=off  InputSameDT=off
  Out1 : Outport
  wires:
  Sum1/1 -> Switch2/3
  Switch2/1 -> Switch1/3
  Compare To Constant1/1 -> Switch2/2
  Switch/1 -> Switch1/1
  Sum/1 -> Switch/3
  Compare To Constant/1 -> Switch/2
  Mod/1 -> Compare To Constant/1, Sum/1, Switch1/2, Switch2/1, Compare To Constant1/1, Sum1/1, Switch/1
  Switch1/1 -> Out1/1  "Mod_rad"
  Constant2/1 -> Sum1/2
  Constant1/1 -> Sum/2
  In1/1 -> Mod/1
  Constant3/1 -> Mod/2

== system Shanthan_Heeirthan_EE469S3D_R45 (1)/S3D_Plant/Comm/P3/DirectionCompensation2 ==
  In1 : Inport
  Compare To Constant : simulink/Logic and Bit Operations/Compare To Constant  relop=<=  const=pi  OutDataTypeStr=boolean
  Compare To Constant1 : simulink/Logic and Bit Operations/Compare To Constant  relop=>=  const=-pi  OutDataTypeStr=boolean
  Constant1 : Constant  Value=2*pi  SampleTime=dt0
  Constant2 : Constant  Value=2*pi  SampleTime=dt0
  Constant3 : Constant  Value=2*pi  SampleTime=dt0
  Mod : Math  Operator=mod
  Sum : Sum  Inputs=|+-
  Sum1 : Sum  Inputs=|++
  Switch : Switch  Criteria=u2 > Threshold  SaturateOnIntegerOverflow=off  InputSameDT=off
  Switch1 : Switch  SaturateOnIntegerOverflow=off  InputSameDT=off
  Switch2 : Switch  Criteria=u2 > Threshold  SaturateOnIntegerOverflow=off  InputSameDT=off
  Out1 : Outport
  wires:
  Sum1/1 -> Switch2/3
  Switch2/1 -> Switch1/3
  Compare To Constant1/1 -> Switch2/2
  Switch/1 -> Switch1/1
  Sum/1 -> Switch/3
  Compare To Constant/1 -> Switch/2
  Mod/1 -> Compare To Constant/1, Sum/1, Switch1/2, Switch2/1, Compare To Constant1/1, Sum1/1, Switch/1
  Switch1/1 -> Out1/1  "Mod_rad"
  Constant2/1 -> Sum1/2
  Constant1/1 -> Sum/2
  In1/1 -> Mod/1
  Constant3/1 -> Mod/2

== system Shanthan_Heeirthan_EE469S3D_R45 (1)/S3D_Plant/Comm/P4/DirectionCompensation2 ==
  In1 : Inport
  Compare To Constant : simulink/Logic and Bit Operations/Compare To Constant  relop=<=  const=pi  OutDataTypeStr=boolean
  Compare To Constant1 : simulink/Logic and Bit Operations/Compare To Constant  relop=>=  const=-pi  OutDataTypeStr=boolean
  Constant1 : Constant  Value=2*pi  SampleTime=dt0
  Constant2 : Constant  Value=2*pi  SampleTime=dt0
  Constant3 : Constant  Value=2*pi  SampleTime=dt0
  Mod : Math  Operator=mod
  Sum : Sum  Inputs=|+-
  Sum1 : Sum  Inputs=|++
  Switch : Switch  Criteria=u2 > Threshold  SaturateOnIntegerOverflow=off  InputSameDT=off
  Switch1 : Switch  SaturateOnIntegerOverflow=off  InputSameDT=off
  Switch2 : Switch  Criteria=u2 > Threshold  SaturateOnIntegerOverflow=off  InputSameDT=off
  Out1 : Outport
  wires:
  Sum1/1 -> Switch2/3
  Switch2/1 -> Switch1/3
  Compare To Constant1/1 -> Switch2/2
  Switch/1 -> Switch1/1
  Sum/1 -> Switch/3
  Compare To Constant/1 -> Switch/2
  Mod/1 -> Compare To Constant/1, Sum/1, Switch1/2, Switch2/1, Compare To Constant1/1, Sum1/1, Switch/1
  Switch1/1 -> Out1/1  "Mod_rad"
  Constant2/1 -> Sum1/2
  Constant1/1 -> Sum/2
  In1/1 -> Mod/1
  Constant3/1 -> Mod/2

== system Shanthan_Heeirthan_EE469S3D_R45 (1)/S3D_Plant/Integrate/CentroidData/FindCentroid ==
  MP : Inport
  XCG : Inport  Port=2
  Bus Selector1 : BusSelector  OutputSignals=x_m
  Bus Selector{6..7,9..10} (4 alike) : BusSelector  OutputSignals=tht_rad
  Bus Selector2 : BusSelector  OutputSignals=y_m
  Bus Selector5 : BusSelector  OutputSignals=Xcg_m,Ycg_m
  Bus Selector8 : BusSelector  OutputSignals=Xcg_m,Ycg_m
  Product{2..5} (4 alike) : Product
  Sum1 : Sum  Inputs=|+-
  Sum2 : Sum  Inputs=|+-
  Sum3 : Sum  Inputs=|++
  Sum4 : Sum  Inputs=|+-
  Trigonometric Function2 : Trigonometry
  Trigonometric Function3 : Trigonometry  Operator=cos
  Trigonometric Function4 : Trigonometry  Operator=cos
  Trigonometric Function5 : Trigonometry
  Xcentroid : Outport
  Ycentroid : Outport  Port=2
  wires:
  Bus Selector2/1 -> Sum4/1  "<y_m>"
  Sum2/1 -> Sum1/2
  Bus Selector7/1 -> Trigonometric Function2/1  "<tht_rad>"
  Trigonometric Function4/1 -> Product5/2
  Bus Selector8/2 -> Product5/1  "<Ycg_m>"
  Bus Selector8/1 -> Product4/2  "<Xcg_m>"
  Product5/1 -> Sum3/2
  Bus Selector9/1 -> Trigonometric Function5/1  "<tht_rad>"
  Product4/1 -> Sum3/1
  Bus Selector1/1 -> Sum1/1  "<x_m>"
  Sum1/1 -> Xcentroid/1  "x_m"
  Trigonometric Function3/1 -> Product2/1
  Product3/1 -> Sum2/2
  Bus Selector5/2 -> Product3/1  "<Ycg_m>"
  Bus Selector6/1 -> Trigonometric Function3/1  "<tht_rad>"
  Product2/1 -> Sum2/1
  Bus Selector10/1 -> Trigonometric Function4/1  "<tht_rad>"
  Trigonometric Function5/1 -> Product4/1
  Bus Selector5/1 -> Product2/2  "<Xcg_m>"
  Trigonometric Function2/1 -> Product3/2
  XCG/1 -> Bus Selector10/1, Bus Selector9/1, Bus Selector2/1, Bus Selector7/1, Bus Selector1/1, Bus Selector6/1
  MP/1 -> Bus Selector5/1, Bus Selector8/1
  Sum4/1 -> Ycentroid/1  "y_m"
  Sum3/1 -> Sum4/2

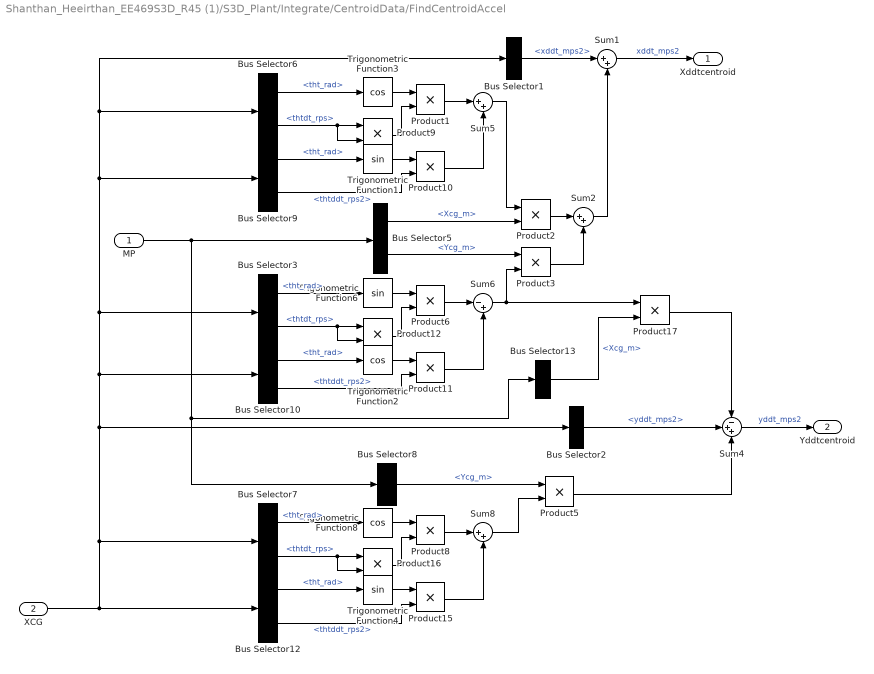
== system Shanthan_Heeirthan_EE469S3D_R45 (1)/S3D_Plant/Integrate/CentroidData/FindCentroidAccel ==
  MP : Inport
  XCG : Inport  Port=2
  Bus Selector1 : BusSelector  OutputSignals=xddt_mps2
  Bus Selector10 : BusSelector  OutputSignals=tht_rad,thtddt_rps2
  Bus Selector12 : BusSelector  OutputSignals=tht_rad,thtddt_rps2
  Bus Selector13 : BusSelector  OutputSignals=Xcg_m
  Bus Selector2 : BusSelector  OutputSignals=yddt_mps2
  Bus Selector3 : BusSelector  OutputSignals=tht_rad,thtdt_rps
  Bus Selector5 : BusSelector  OutputSignals=Xcg_m,Ycg_m
  Bus Selector6 : BusSelector  OutputSignals=tht_rad,thtdt_rps
  Bus Selector7 : BusSelector  OutputSignals=tht_rad,thtdt_rps
  Bus Selector8 : BusSelector  OutputSignals=Ycg_m
  Bus Selector9 : BusSelector  OutputSignals=tht_rad,thtddt_rps2
  Product{1..3,5..6,8..12,15..17} (13 alike) : Product
  Sum{1..2,5,8} (4 alike) : Sum  Inputs=|++
  Sum4 : Sum  Inputs=-++
  Sum6 : Sum  Inputs=|-+
  Trigonometric Function1 : Trigonometry
  Trigonometric Function2 : Trigonometry  Operator=cos
  Trigonometric Function3 : Trigonometry  Operator=cos
  Trigonometric Function4 : Trigonometry
  Trigonometric Function6 : Trigonometry
  Trigonometric Function8 : Trigonometry  Operator=cos
  Xddtcentroid : Outport
  Yddtcentroid : Outport  Port=2
  wires:
  Sum8/1 -> Product5/2
  Product15/1 -> Sum8/2
  Product8/1 -> Sum8/1
  Bus Selector12/2 -> Product15/2  "<thtddt_rps2>"
  Bus Selector12/1 -> Trigonometric Function4/1  "<tht_rad>"
  Trigonometric Function4/1 -> Product15/1
  Product16/1 -> Product8/2
  Bus Selector7/2 -> Product16/1, Product16/2  "<thtdt_rps>"
  Bus Selector7/1 -> Trigonometric Function8/1  "<tht_rad>"
  Trigonometric Function8/1 -> Product8/1
  Sum6/1 -> Product17/1, Product3/2
  Product11/1 -> Sum6/2
  Product6/1 -> Sum6/1
  Bus Selector10/2 -> Product11/2  "<thtddt_rps2>"
  Bus Selector10/1 -> Trigonometric Function2/1  "<tht_rad>"
  Trigonometric Function2/1 -> Product11/1
  Product12/1 -> Product6/2
  Bus Selector3/2 -> Product12/1, Product12/2  "<thtdt_rps>"
  Bus Selector3/1 -> Trigonometric Function6/1  "<tht_rad>"
  Trigonometric Function6/1 -> Product6/1
  Sum5/1 -> Product2/1
  Product10/1 -> Sum5/2
  Product1/1 -> Sum5/1
  Bus Selector9/2 -> Product10/2  "<thtddt_rps2>"
  Bus Selector9/1 -> Trigonometric Function1/1  "<tht_rad>"
  Trigonometric Function1/1 -> Product10/1
  Product9/1 -> Product1/2
  Bus Selector6/2 -> Product9/1, Product9/2  "<thtdt_rps>"
  Bus Selector2/1 -> Sum4/2  "<yddt_mps2>"
  Sum2/1 -> Sum1/2
  Bus Selector1/1 -> Sum1/1  "<xddt_mps2>"
  Sum1/1 -> Xddtcentroid/1  "xddt_mps2"
  Product3/1 -> Sum2/2
  Bus Selector6/1 -> Trigonometric Function3/1  "<tht_rad>"
  Product2/1 -> Sum2/1
  XCG/1 -> Bus Selector12/1, Bus Selector1/1, Bus Selector6/1, Bus Selector9/1, Bus Selector3/1, Bus Selector10/1, Bus Selector2/1, Bus Selector7/1
  MP/1 -> Bus Selector8/1, Bus Selector13/1, Bus Selector5/1
  Sum4/1 -> Yddtcentroid/1  "yddt_mps2"
  Product5/1 -> Sum4/3
  Trigonometric Function3/1 -> Product1/1
  Bus Selector5/1 -> Product2/2  "<Xcg_m>"
  Bus Selector5/2 -> Product3/1  "<Ycg_m>"
  Bus Selector8/1 -> Product5/1  "<Ycg_m>"
  Bus Selector13/1 -> Product17/2  "<Xcg_m>"
  Product17/1 -> Sum4/1

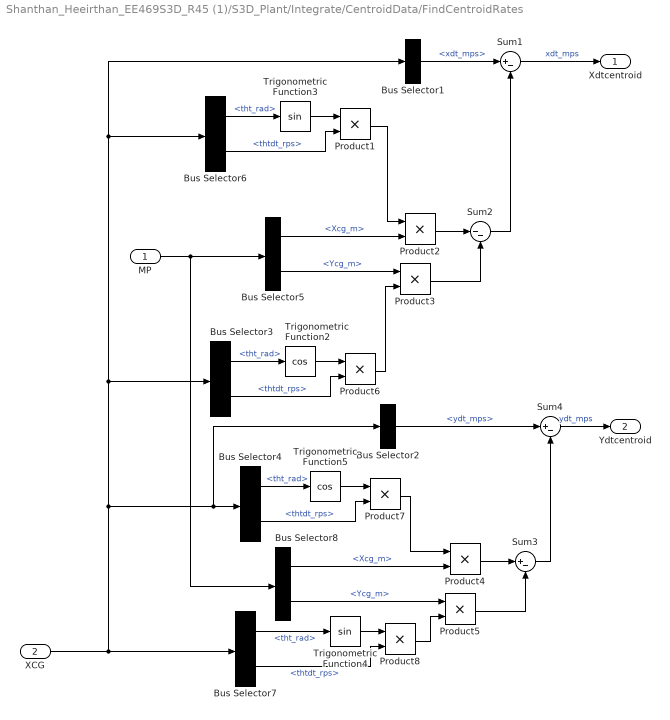
== system Shanthan_Heeirthan_EE469S3D_R45 (1)/S3D_Plant/Integrate/CentroidData/FindCentroidRates ==
  MP : Inport
  XCG : Inport  Port=2
  Bus Selector1 : BusSelector  OutputSignals=xdt_mps
  Bus Selector2 : BusSelector  OutputSignals=ydt_mps
  Bus Selector{3..4,6..7} (4 alike) : BusSelector  OutputSignals=tht_rad,thtdt_rps
  Bus Selector5 : BusSelector  OutputSignals=Xcg_m,Ycg_m
  Bus Selector8 : BusSelector  OutputSignals=Xcg_m,Ycg_m
  Product{1..8} (8 alike) : Product
  Sum1 : Sum  Inputs=|+-
  Sum2 : Sum  Inputs=|--
  Sum3 : Sum  Inputs=|+-
  Sum4 : Sum  Inputs=|+-
  Trigonometric Function2 : Trigonometry  Operator=cos
  Trigonometric Function3 : Trigonometry
  Trigonometric Function4 : Trigonometry
  Trigonometric Function5 : Trigonometry  Operator=cos
  Xdtcentroid : Outport
  Ydtcentroid : Outport  Port=2
  wires:
  Bus Selector7/2 -> Product8/2  "<thtdt_rps>"
  Product8/1 -> Product5/2
  Trigonometric Function4/1 -> Product8/1
  Bus Selector8/2 -> Product5/1  "<Ycg_m>"
  Bus Selector8/1 -> Product4/2  "<Xcg_m>"
  Bus Selector4/2 -> Product7/2  "<thtdt_rps>"
  Product7/1 -> Product4/1
  Trigonometric Function5/1 -> Product7/1
  Product6/1 -> Product3/2
  Bus Selector5/2 -> Product3/1  "<Ycg_m>"
  Bus Selector3/2 -> Product6/2  "<thtdt_rps>"
  Trigonometric Function2/1 -> Product6/1
  Bus Selector5/1 -> Product2/2  "<Xcg_m>"
  Product1/1 -> Product2/1
  Bus Selector6/2 -> Product1/2  "<thtdt_rps>"
  Trigonometric Function3/1 -> Product1/1
  Sum3/1 -> Sum4/2
  Sum4/1 -> Ydtcentroid/1  "ydt_mps"
  MP/1 -> Bus Selector8/1, Bus Selector5/1
  XCG/1 -> Bus Selector3/1, Bus Selector6/1, Bus Selector1/1, Bus Selector2/1, Bus Selector4/1, Bus Selector7/1
  Bus Selector7/1 -> Trigonometric Function4/1  "<tht_rad>"
  Product2/1 -> Sum2/1
  Bus Selector6/1 -> Trigonometric Function3/1  "<tht_rad>"
  Product3/1 -> Sum2/2
  Sum1/1 -> Xdtcentroid/1  "xdt_mps"
  Bus Selector1/1 -> Sum1/1  "<xdt_mps>"
  Product4/1 -> Sum3/1
  Bus Selector4/1 -> Trigonometric Function5/1  "<tht_rad>"
  Product5/1 -> Sum3/2
  Bus Selector3/1 -> Trigonometric Function2/1  "<tht_rad>"
  Sum2/1 -> Sum1/2
  Bus Selector2/1 -> Sum4/1  "<ydt_mps>"

== system Shanthan_Heeirthan_EE469S3D_R45 (1)/S3D_Plant/MassProperties/GetCGnJ/Subsystem ==
  Xmom : Inport
  Ymom : Inport  Port=2
  M_kg : Inport  Port=3
  Product : Product  Inputs=*/
  Product1 : Product  Inputs=*/
  Product2 : Product
  Product3 : Product
  Product4 : Product
  Sum : Sum  Inputs=|++
  Jpat : Outport
  Xcg : Outport  Port=2
  Ycg : Outport  Port=3
  wires:
  Product4/1 -> Jpat/1  "Jpat_kgm2"
  M_kg/1 -> Product/2, Product1/2, Product4/2
  Sum/1 -> Product4/1
  Product3/1 -> Sum/2
  Product2/1 -> Sum/1
  Xmom/1 -> Product/1
  Ymom/1 -> Product1/1
  Product/1 -> Xcg/1, Product2/2, Product2/1  "Xcg_m"
  Product1/1 -> Ycg/1, Product3/1, Product3/2  "Ycg_m"

== system Shanthan_Heeirthan_EE469S3D_R45 (1)/S3D_Plant/OutputDataProcessing/MakePlot/MakePlot ==
  PlotData : Inport
  Interpreted MATLAB Function : MATLABFcn  MATLABFcn=PlotS3D  SampleTime=dt0*fr
  Rate Transition : RateTransition  InitialCondition=[zeros(11,1);0.1*[M1;M2;M3;M4];PTvec;zeros(8,1);0;zeros(8,1);zeros(9,1)]  OutPortSampleTime=dt0*fr
  Terminator : Terminator
  wires:
  PlotData/1 -> Rate Transition/1
  Interpreted MATLAB Function/1 -> Terminator/1
  Rate Transition/1 -> Interpreted MATLAB Function/1

== system Shanthan_Heeirthan_EE469S3D_R45 (1)/S3D_Plant/Sensors/CASE1/THTaccel ==
  X : Inport
  Abs : Abs  SaturateOnIntegerOverflow=off
  Bus Selector3 : BusSelector  OutputSignals=thtddt_rps2
  CURRENT : Subsystem  TreatAsAtomicUnit=on
  Compare To Constant : simulink/Logic and Bit Operations/Compare To Constant  relop=<=  const=0.5  OutDataTypeStr=boolean
  Constant1 : Constant  Value=LVL.Sfail(9)  SampleTime=dt0
  Constant2 : Constant  Value=LVL.Sft(9,1)+rand*(LVL.Sft(9,2)-LVL.Sft(9,1))  SampleTime=dt0
  Digital Clock : DigitalClock  SampleTime=dt0
  Gain : Gain  Gain=LVL.SN
  Gain4 : Gain  Gain=r2d
  If : If  IfExpression=u1 < -0.5  ElseIfExpressions=u1 > 0.5 & u1 < 1.5
  Logical Operator : Logic  Operator=OR  AllPortsSameDT=off  OutDataTypeStr=boolean
  MAX : Subsystem  TreatAsAtomicUnit=on
  MIN : Subsystem  TreatAsAtomicUnit=on
  Merge : Merge  Inputs=3
  Quantizer : Quantizer  QuantizationInterval=SQ(9)  SampleTime=dt0
  Random Number : RandomNumber  Variance=LVL.SigSense(9)  Seed=9  SampleTime=dt0
  Relational Operator : RelationalOperator  Operator=<  OutDataTypeStr=boolean  InputSameDT=off
  Saturation : Saturate  UpperLimit=SLIM(9,2)  LowerLimit=SLIM(9,1)
  Sum : Sum  Inputs=|++
  Switch : Switch  Criteria=u2 > Threshold  SaturateOnIntegerOverflow=off  InputSameDT=off
  Unit Delay : UnitDelay  SampleTime=dt0  HasFrameUpgradeWarning=on
  thtddt1 : Outport
  wires:
  Saturation/1 -> Quantizer/1
  Quantizer/1 -> Unit Delay/1, thtddt1/1
  Gain4/1 -> Sum/1
  Compare To Constant/1 -> Logical Operator/2
  Abs/1 -> Compare To Constant/1
  Constant1/1 -> If/1, Abs/1
  Logical Operator/1 -> Switch/2
  Relational Operator/1 -> Logical Operator/1
  Sum/1 -> Switch/1
  Bus Selector3/1 -> Gain4/1  "<thtddt_rps2>"
  Gain/1 -> Sum/2
  Random Number/1 -> Gain/1
  Merge/1 -> Switch/3
  MIN/1(Out1) -> Merge/1
  CURRENT/1(Out1) -> Merge/3
  X/1 -> Bus Selector3/1
  Constant2/1 -> Relational Operator/2
  MAX/1(Out1) -> Merge/2
  Unit Delay/1 -> CURRENT/1(In1)
  If/3 -> CURRENT/Action
  Digital Clock/1 -> Relational Operator/1
  Switch/1 -> Saturation/1
  If/2 -> MAX/Action
  If/1 -> MIN/Action

== system Shanthan_Heeirthan_EE469S3D_R45 (1)/S3D_Plant/Sensors/CASE1/THTpos1 ==
  X : Inport
  Abs : Abs  SaturateOnIntegerOverflow=off
  Bus Selector3 : BusSelector  OutputSignals=tht_rad
  CURRENT : Subsystem  TreatAsAtomicUnit=on
  Compare To Constant : simulink/Logic and Bit Operations/Compare To Constant  relop=<=  const=0.5  OutDataTypeStr=boolean
  Constant1 : Constant  Value=LVL.Sfail(7)  SampleTime=dt0
  Constant2 : Constant  Value=LVL.Sft(7,1)+rand*(LVL.Sft(7,2)-LVL.Sft(7,1))  SampleTime=dt0
  Digital Clock : DigitalClock  SampleTime=dt0
  Gain : Gain  Gain=LVL.SN
  Gain4 : Gain  Gain=r2d
  If : If  IfExpression=u1 < -0.5  ElseIfExpressions=u1 > 0.5 & u1 < 1.5
  Logical Operator : Logic  Operator=OR  AllPortsSameDT=off  OutDataTypeStr=boolean
  MAX : Subsystem  TreatAsAtomicUnit=on
  MIN : Subsystem  TreatAsAtomicUnit=on
  Merge : Merge  Inputs=3
  Quantizer : Quantizer  QuantizationInterval=SQ(7)  SampleTime=dt0
  Random Number : RandomNumber  Variance=LVL.SigSense(7)  Seed=7  SampleTime=dt0
  Relational Operator : RelationalOperator  Operator=<  OutDataTypeStr=boolean  InputSameDT=off
  Saturation : Saturate  UpperLimit=SLIM(7,2)  LowerLimit=SLIM(7,1)
  Sum : Sum  Inputs=|++
  Switch : Switch  Criteria=u2 > Threshold  SaturateOnIntegerOverflow=off  InputSameDT=off
  Unit Delay : UnitDelay  SampleTime=dt0  HasFrameUpgradeWarning=on
  tht1 : Outport
  wires:
  Saturation/1 -> Quantizer/1
  Switch/1 -> Saturation/1
  Quantizer/1 -> tht1/1, Unit Delay/1
  Gain4/1 -> Sum/1
  Compare To Constant/1 -> Logical Operator/2
  Abs/1 -> Compare To Constant/1
  Constant1/1 -> If/1, Abs/1
  Logical Operator/1 -> Switch/2
  Relational Operator/1 -> Logical Operator/1
  Sum/1 -> Switch/1
  Bus Selector3/1 -> Gain4/1  "<tht_rad>"
  Gain/1 -> Sum/2
  Random Number/1 -> Gain/1
  Merge/1 -> Switch/3
  MIN/1(Out1) -> Merge/1
  CURRENT/1(Out1) -> Merge/3
  X/1 -> Bus Selector3/1
  Constant2/1 -> Relational Operator/2
  MAX/1(Out1) -> Merge/2
  Unit Delay/1 -> CURRENT/1(In1)
  If/3 -> CURRENT/Action
  Digital Clock/1 -> Relational Operator/1
  If/2 -> MAX/Action
  If/1 -> MIN/Action

== system Shanthan_Heeirthan_EE469S3D_R45 (1)/S3D_Plant/Sensors/CASE1/THTvel ==
  X : Inport
  Abs : Abs  SaturateOnIntegerOverflow=off
  Bus Selector3 : BusSelector  OutputSignals=thtdt_rps
  CURRENT : Subsystem  TreatAsAtomicUnit=on
  Compare To Constant : simulink/Logic and Bit Operations/Compare To Constant  relop=<=  const=0.5  OutDataTypeStr=boolean
  Constant1 : Constant  Value=LVL.Sfail(8)  SampleTime=dt0
  Constant2 : Constant  Value=LVL.Sft(8,1)+rand*(LVL.Sft(8,2)-LVL.Sft(8,1))  SampleTime=dt0
  Digital Clock : DigitalClock  SampleTime=dt0
  Gain : Gain  Gain=LVL.SN
  Gain4 : Gain  Gain=r2d
  If : If  IfExpression=u1 < -0.5  ElseIfExpressions=u1 > 0.5 & u1 < 1.5
  Logical Operator : Logic  Operator=OR  AllPortsSameDT=off  OutDataTypeStr=boolean
  MAX : Subsystem  TreatAsAtomicUnit=on
  MIN : Subsystem  TreatAsAtomicUnit=on
  Merge : Merge  Inputs=3
  Quantizer : Quantizer  QuantizationInterval=SQ(8)  SampleTime=dt0
  Random Number : RandomNumber  Variance=LVL.SigSense(8)  Seed=8  SampleTime=dt0
  Relational Operator : RelationalOperator  Operator=<  OutDataTypeStr=boolean  InputSameDT=off
  Saturation : Saturate  UpperLimit=SLIM(8,2)  LowerLimit=SLIM(8,1)
  Sum : Sum  Inputs=|++
  Switch : Switch  Criteria=u2 > Threshold  SaturateOnIntegerOverflow=off  InputSameDT=off
  Unit Delay : UnitDelay  SampleTime=dt0  HasFrameUpgradeWarning=on
  thtdt1 : Outport
  wires:
  Saturation/1 -> Quantizer/1
  Quantizer/1 -> thtdt1/1, Unit Delay/1
  Gain4/1 -> Sum/1
  If/1 -> MIN/Action
  If/2 -> MAX/Action
  Switch/1 -> Saturation/1
  Digital Clock/1 -> Relational Operator/1
  If/3 -> CURRENT/Action
  Unit Delay/1 -> CURRENT/1(In1)
  MAX/1(Out1) -> Merge/2
  Constant2/1 -> Relational Operator/2
  X/1 -> Bus Selector3/1
  CURRENT/1(Out1) -> Merge/3
  MIN/1(Out1) -> Merge/1
  Merge/1 -> Switch/3
  Random Number/1 -> Gain/1
  Gain/1 -> Sum/2
  Bus Selector3/1 -> Gain4/1  "<thtdt_rps>"
  Sum/1 -> Switch/1
  Relational Operator/1 -> Logical Operator/1
  Logical Operator/1 -> Switch/2
  Constant1/1 -> Abs/1, If/1
  Abs/1 -> Compare To Constant/1
  Compare To Constant/1 -> Logical Operator/2

== system Shanthan_Heeirthan_EE469S3D_R45 (1)/S3D_Plant/Sensors/CASE1/Xaccel ==
  X : Inport
  Abs : Abs  SaturateOnIntegerOverflow=off
  Bus Selector3 : BusSelector  OutputSignals=xddt_mps2
  CURRENT : Subsystem  TreatAsAtomicUnit=on
  Compare To Constant : simulink/Logic and Bit Operations/Compare To Constant  relop=<=  const=0.5  OutDataTypeStr=boolean
  Constant1 : Constant  Value=LVL.Sfail(3)  SampleTime=dt0
  Constant2 : Constant  Value=LVL.Sft(3,1)+rand*(LVL.Sft(3,2)-LVL.Sft(3,1))  SampleTime=dt0
  Digital Clock : DigitalClock  SampleTime=dt0
  Gain : Gain  Gain=LVL.SN
  If : If  IfExpression=u1 < -0.5  ElseIfExpressions=u1 > 0.5 & u1 < 1.5
  Logical Operator : Logic  Operator=OR  AllPortsSameDT=off  OutDataTypeStr=boolean
  MAX : Subsystem  TreatAsAtomicUnit=on
  MIN : Subsystem  TreatAsAtomicUnit=on
  Merge : Merge  Inputs=3
  Quantizer : Quantizer  QuantizationInterval=SQ(3)  SampleTime=dt0
  Random Number : RandomNumber  Variance=LVL.SigSense(3)  Seed=3  SampleTime=dt0
  Relational Operator : RelationalOperator  Operator=<  OutDataTypeStr=boolean  InputSameDT=off
  Saturation : Saturate  UpperLimit=SLIM(3,2)  LowerLimit=SLIM(3,1)
  Sum : Sum  Inputs=|++
  Switch : Switch  Criteria=u2 > Threshold  SaturateOnIntegerOverflow=off  InputSameDT=off
  Unit Delay : UnitDelay  SampleTime=dt0  HasFrameUpgradeWarning=on
  xddt1 : Outport
  wires:
  Saturation/1 -> Quantizer/1
  Quantizer/1 -> Unit Delay/1, xddt1/1
  Compare To Constant/1 -> Logical Operator/2
  Abs/1 -> Compare To Constant/1
  Constant1/1 -> If/1, Abs/1
  Logical Operator/1 -> Switch/2
  Relational Operator/1 -> Logical Operator/1
  Sum/1 -> Switch/1
  Bus Selector3/1 -> Sum/1  "<xddt_mps2>"
  Gain/1 -> Sum/2
  Random Number/1 -> Gain/1
  Merge/1 -> Switch/3
  MIN/1(Out1) -> Merge/1
  CURRENT/1(Out1) -> Merge/3
  X/1 -> Bus Selector3/1
  Constant2/1 -> Relational Operator/2
  MAX/1(Out1) -> Merge/2
  Unit Delay/1 -> CURRENT/1(In1)
  If/3 -> CURRENT/Action
  Digital Clock/1 -> Relational Operator/1
  Switch/1 -> Saturation/1
  If/2 -> MAX/Action
  If/1 -> MIN/Action

== system Shanthan_Heeirthan_EE469S3D_R45 (1)/S3D_Plant/Sensors/CASE1/Xpos1 ==
  X : Inport
  Abs : Abs  SaturateOnIntegerOverflow=off
  Bus Selector3 : BusSelector  OutputSignals=x_m
  CURRENT : Subsystem  TreatAsAtomicUnit=on
  Compare To Constant : simulink/Logic and Bit Operations/Compare To Constant  relop=<=  const=0.5  OutDataTypeStr=boolean
  Constant1 : Constant  Value=LVL.Sfail(1)  SampleTime=dt0
  Constant2 : Constant  Value=LVL.Sft(1,1)+rand*(LVL.Sft(1,2)-LVL.Sft(1,1))  SampleTime=dt0
  Digital Clock : DigitalClock  SampleTime=dt0
  Gain : Gain  Gain=LVL.SN
  If : If  IfExpression=u1 < -0.5  ElseIfExpressions=u1 > 0.5 & u1 < 1.5
  Logical Operator : Logic  Operator=OR  AllPortsSameDT=off  OutDataTypeStr=boolean
  MAX : Subsystem  TreatAsAtomicUnit=on
  MIN : Subsystem  TreatAsAtomicUnit=on
  Merge : Merge  Inputs=3
  Quantizer : Quantizer  QuantizationInterval=SQ(1)  SampleTime=dt0
  Random Number : RandomNumber  Variance=LVL.SigSense(1)  Seed=1  SampleTime=dt0
  Relational Operator : RelationalOperator  Operator=<  OutDataTypeStr=boolean  InputSameDT=off
  Saturation : Saturate  UpperLimit=SLIM(1,2)  LowerLimit=SLIM(1,1)
  Sum : Sum  Inputs=|++
  Switch : Switch  Criteria=u2 > Threshold  SaturateOnIntegerOverflow=off  InputSameDT=off
  Unit Delay : UnitDelay  SampleTime=dt0  HasFrameUpgradeWarning=on
  x1 : Outport
  wires:
  Saturation/1 -> Quantizer/1
  Quantizer/1 -> Unit Delay/1, x1/1
  Compare To Constant/1 -> Logical Operator/2
  Abs/1 -> Compare To Constant/1
  Constant1/1 -> If/1, Abs/1
  Logical Operator/1 -> Switch/2
  Relational Operator/1 -> Logical Operator/1
  Sum/1 -> Switch/1
  Bus Selector3/1 -> Sum/1  "<x_m>"
  Gain/1 -> Sum/2
  Random Number/1 -> Gain/1
  Merge/1 -> Switch/3
  MIN/1(Out1) -> Merge/1
  CURRENT/1(Out1) -> Merge/3
  X/1 -> Bus Selector3/1
  Constant2/1 -> Relational Operator/2
  MAX/1(Out1) -> Merge/2
  Unit Delay/1 -> CURRENT/1(In1)
  If/3 -> CURRENT/Action
  Digital Clock/1 -> Relational Operator/1
  Switch/1 -> Saturation/1
  If/2 -> MAX/Action
  If/1 -> MIN/Action

== system Shanthan_Heeirthan_EE469S3D_R45 (1)/S3D_Plant/Sensors/CASE1/Xvel ==
  X : Inport
  Abs : Abs  SaturateOnIntegerOverflow=off
  Bus Selector3 : BusSelector  OutputSignals=xdt_mps
  CURRENT : Subsystem  TreatAsAtomicUnit=on
  Compare To Constant : simulink/Logic and Bit Operations/Compare To Constant  relop=<=  const=0.5  OutDataTypeStr=boolean
  Constant1 : Constant  Value=LVL.Sfail(2)  SampleTime=dt0
  Constant2 : Constant  Value=LVL.Sft(2,1)+rand*(LVL.Sft(2,2)-LVL.Sft(2,1))  SampleTime=dt0
  Digital Clock : DigitalClock  SampleTime=dt0
  Gain : Gain  Gain=LVL.SN
  If : If  IfExpression=u1 < -0.5  ElseIfExpressions=u1 > 0.5 & u1 < 1.5
  Logical Operator : Logic  Operator=OR  AllPortsSameDT=off  OutDataTypeStr=boolean
  MAX : Subsystem  TreatAsAtomicUnit=on
  MIN : Subsystem  TreatAsAtomicUnit=on
  Merge : Merge  Inputs=3
  Quantizer : Quantizer  QuantizationInterval=SQ(2)  SampleTime=dt0
  Random Number : RandomNumber  Variance=LVL.SigSense(2)  Seed=2  SampleTime=dt0
  Relational Operator : RelationalOperator  Operator=<  OutDataTypeStr=boolean  InputSameDT=off
  Saturation : Saturate  UpperLimit=SLIM(2,2)  LowerLimit=SLIM(2,1)
  Sum : Sum  Inputs=|++
  Switch : Switch  Criteria=u2 > Threshold  SaturateOnIntegerOverflow=off  InputSameDT=off
  Unit Delay : UnitDelay  SampleTime=dt0  HasFrameUpgradeWarning=on
  xdt1 : Outport
  wires:
  Saturation/1 -> Quantizer/1
  Quantizer/1 -> xdt1/1, Unit Delay/1
  If/1 -> MIN/Action
  If/2 -> MAX/Action
  Switch/1 -> Saturation/1
  Digital Clock/1 -> Relational Operator/1
  If/3 -> CURRENT/Action
  Unit Delay/1 -> CURRENT/1(In1)
  MAX/1(Out1) -> Merge/2
  Constant2/1 -> Relational Operator/2
  X/1 -> Bus Selector3/1
  CURRENT/1(Out1) -> Merge/3
  MIN/1(Out1) -> Merge/1
  Merge/1 -> Switch/3
  Random Number/1 -> Gain/1
  Gain/1 -> Sum/2
  Bus Selector3/1 -> Sum/1  "<xdt_mps>"
  Sum/1 -> Switch/1
  Relational Operator/1 -> Logical Operator/1
  Logical Operator/1 -> Switch/2
  Constant1/1 -> Abs/1, If/1
  Abs/1 -> Compare To Constant/1
  Compare To Constant/1 -> Logical Operator/2
